simulink model "DynamicModel"  (R2018a)
settings: Solver=VariableStepAuto  StartTime=0.0  StopTime=10.0  RelTol=1e-3
model workspace (MAT data in the model file):
  Iz = 0.05807429185
  cf = 50000
  cr = 50000
  k1 = 2
  k2 = 5
  k3 = 3
  k4 = 6
  lf = 0.16002
  lr = 0.16002
  m = 2.26796
libraries: templibrary x1, dspmathops x1
settings Model: Creator=aswerdlow  LastModifiedBy=aswerdlow

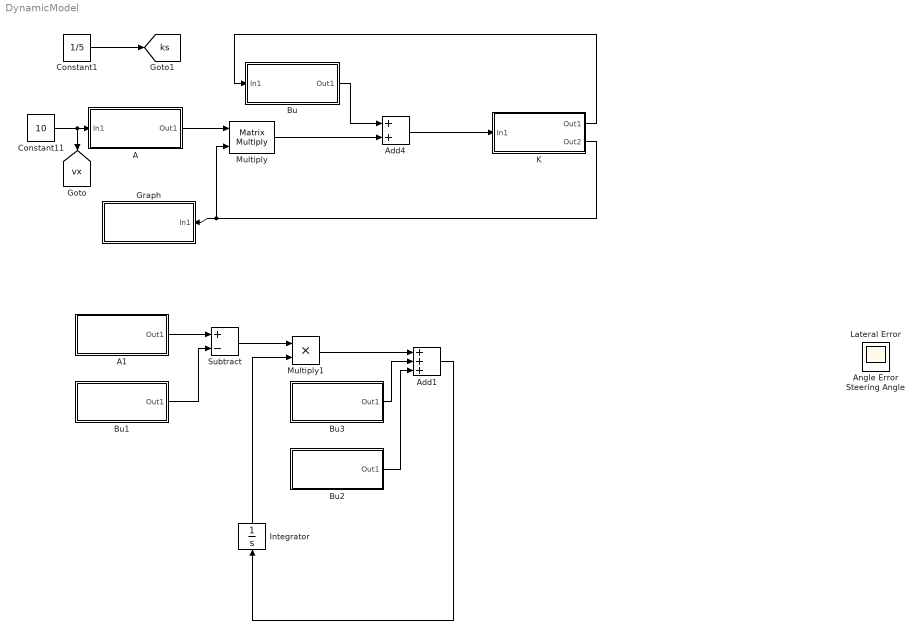
== system DynamicModel ==
  A : Subsystem
  A1 : Subsystem
  Add1 : Sum  Inputs=+++
  Add4 : Sum
  Bu : Subsystem
  Bu1 : Subsystem
  Bu2 : Subsystem
  Bu3 : Subsystem
  Constant1 : Constant  Value=1/5
  Constant11 : Constant  Value=10
  Graph : Subsystem
  Integrator : Integrator
  K : Subsystem
  Multiply : Product  Multiplication=Matrix(*)
  Multiply1 : Product
  Subtract : Sum  Inputs=+-
  Angle Error : Scope
  Lateral Error : Scope
  Steering Angle : Scope
  tag scope: ks=global, vx=global
  wires:
  Constant11/1 -> A/1(In1), [vx]
  A/1(Out1) -> Multiply/1
  Multiply/1 -> Add4/2
  Bu/1(Out1) -> Add4/1
  Add4/1 -> K/1(In1)
  K/1(Out1) -> Bu/1(In1)
  K/2(Out2) -> Graph/1(In1), Multiply/2
  Constant1/1 -> [ks]
  Subtract/1 -> Multiply1/1
  Bu1/1(Out1) -> Subtract/2
  Multiply1/1 -> Add1/1
  Integrator/1 -> Multiply1/2
  Add1/1 -> Integrator/1
  Bu3/1(Out1) -> Add1/2
  Bu2/1(Out1) -> Add1/3
  A1/1(Out1) -> Subtract/1

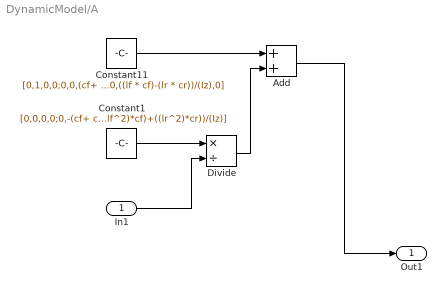
== system DynamicModel/A ==
  In1 : Inport
  Add : Sum
  Constant1 : Constant  Value=[0,0,0,0;0,-(cf+ cr)/(m),0,(lr * cr)-(lf * cf)/(m);0,0,0,0;0,((lr * cr)-(lf * cf))/(Iz),0,-(((lf^2)*cf)+((lr^2)*cr))/(Iz)]  VectorParams1D=off
  Constant11 : Constant  Value=[0,1,0,0;0,0,(cf+ cr)/(m),0;0,0,0,1;0,0,((lf * cf)-(lr * cr))/(Iz),0]  VectorParams1D=off
  Divide : Product  Inputs=*/
  Out1 : Outport
  wires:
  In1/1 -> Divide/2
  Constant11/1 -> Add/1
  Constant1/1 -> Divide/1
  Divide/1 -> Add/2
  Add/1 -> Out1/1

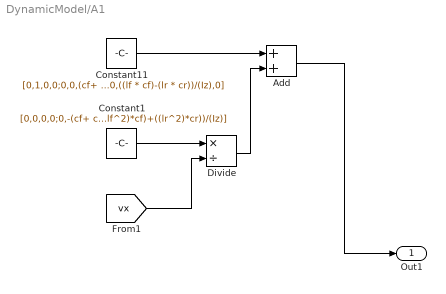
== system DynamicModel/A1 ==
  Add : Sum
  Constant1 : Constant  Value=[0,0,0,0;0,-(cf+ cr)/(m),0,(lr * cr)-(lf * cf)/(m);0,0,0,0;0,((lr * cr)-(lf * cf))/(Iz),0,-(((lf^2)*cf)+((lr^2)*cr))/(Iz)]  VectorParams1D=off
  Constant11 : Constant  Value=[0,1,0,0;0,0,(cf+ cr)/(m),0;0,0,0,1;0,0,((lf * cf)-(lr * cr))/(Iz),0]  VectorParams1D=off
  Divide : Product  Inputs=*/
  Out1 : Outport
  wires:
  [vx] -> Divide/2
  Constant11/1 -> Add/1
  Constant1/1 -> Divide/1
  Divide/1 -> Add/2
  Add/1 -> Out1/1

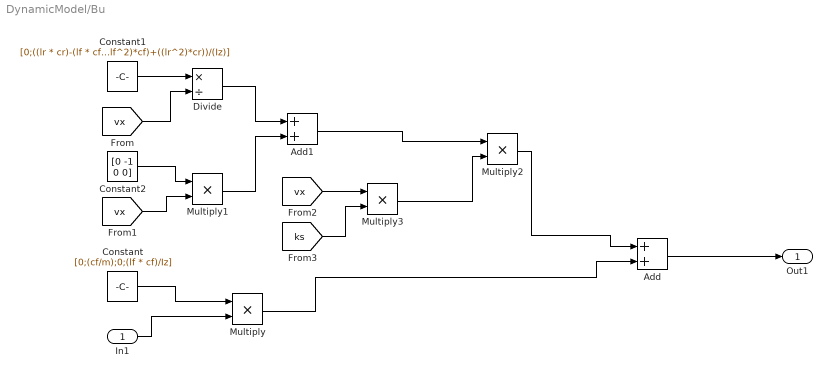
== system DynamicModel/Bu ==
  In1 : Inport
  Add : Sum
  Add1 : Sum
  Constant : Constant  Value=[0;(cf/m);0;(lf * cf)/Iz]  VectorParams1D=off
  Constant1 : Constant  Value=[0;((lr * cr)-(lf * cf))/m;0;-(((lf^2)*cf)+((lr^2)*cr))/(Iz)]  VectorParams1D=off
  Constant2 : Constant  Value=[0 -1 0 0]
  Divide : Product  Inputs=*/
  Multiply{,1..3} (4 alike) : Product
  Out1 : Outport
  wires:
  In1/1 -> Multiply/2
  Add/1 -> Out1/1
  Constant/1 -> Multiply/1
  Multiply/1 -> Add/2
  Constant1/1 -> Divide/1
  [vx] -> Divide/2
  Constant2/1 -> Multiply1/1
  [vx] -> Multiply1/2
  Divide/1 -> Add1/1
  Multiply1/1 -> Add1/2
  Add1/1 -> Multiply2/1
  [vx] -> Multiply3/1
  [ks] -> Multiply3/2
  Multiply3/1 -> Multiply2/2
  Multiply2/1 -> Add/1

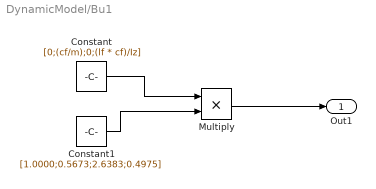
== system DynamicModel/Bu1 ==
  Constant : Constant  Value=[0;(cf/m);0;(lf * cf)/Iz]  VectorParams1D=off
  Constant1 : Constant  Value=[1.0000;0.5673;2.6383;0.4975]  VectorParams1D=off
  Multiply : Product
  Out1 : Outport
  wires:
  Constant1/1 -> Multiply/2
  Multiply/1 -> Out1/1
  Constant/1 -> Multiply/1

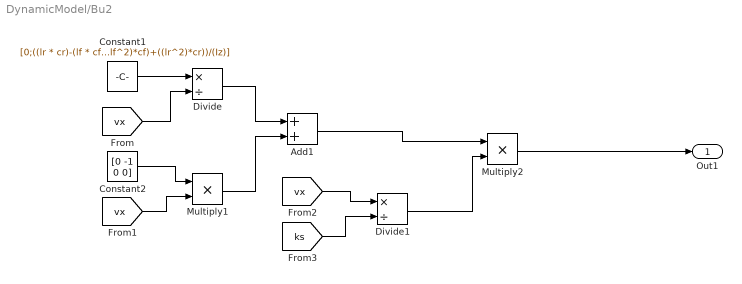
== system DynamicModel/Bu2 ==
  Add1 : Sum
  Constant1 : Constant  Value=[0;((lr * cr)-(lf * cf))/m;0;-(((lf^2)*cf)+((lr^2)*cr))/(Iz)]  VectorParams1D=off
  Constant2 : Constant  Value=[0 -1 0 0]
  Divide : Product  Inputs=*/
  Divide1 : Product  Inputs=*/
  Multiply1 : Product
  Multiply2 : Product
  Out1 : Outport
  wires:
  Multiply2/1 -> Out1/1
  Constant1/1 -> Divide/1
  [vx] -> Divide/2
  Constant2/1 -> Multiply1/1
  [vx] -> Multiply1/2
  Divide/1 -> Add1/1
  Multiply1/1 -> Add1/2
  Add1/1 -> Multiply2/1
  [vx] -> Divide1/1
  [ks] -> Divide1/2
  Divide1/1 -> Multiply2/2

== system DynamicModel/Bu3 ==
  Constant : Constant  Value=[0;(cf/m);0;(lf * cf)/Iz]  VectorParams1D=off
  Multiply : Product
  Subsystem : Subsystem
  Out1 : Outport
  wires:
  Multiply/1 -> Out1/1
  Constant/1 -> Multiply/1
  Subsystem/1(Out1) -> Multiply/2

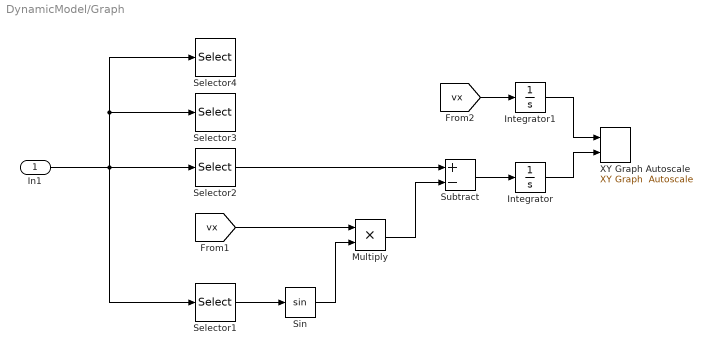
== system DynamicModel/Graph ==
  In1 : Inport
  Integrator : Integrator
  Integrator1 : Integrator
  Multiply : Product
  Selector1 : Selector  InputPortWidth=4  IndexOptions=Index vector (dialog)  Indices=3  OutputSizes=1
  Selector2 : Selector  InputPortWidth=4  IndexOptions=Index vector (dialog)  Indices=2  OutputSizes=1
  Selector3 : Selector  InputPortWidth=4  IndexOptions=Index vector (dialog)  Indices=3  OutputSizes=1
  Selector4 : Selector  InputPortWidth=4  IndexOptions=Index vector (dialog)  Indices=1  OutputSizes=1
  Sin : Trigonometry
  Subtract : Sum  Inputs=+-
  XY Graph Autoscale : templibrary/XY Graph  Autoscale  xmin=-1  xmax=1  ymin=-1  ymax=1  st=-1
  wires:
  Selector2/1 -> Subtract/1
  In1/1 -> Selector3/1, Selector4/1, Selector2/1, Selector1/1
  [vx] -> Multiply/1
  Sin/1 -> Multiply/2
  Selector1/1 -> Sin/1
  Multiply/1 -> Subtract/2
  Subtract/1 -> Integrator/1
  [vx] -> Integrator1/1
  Integrator1/1 -> XY Graph Autoscale/1
  Integrator/1 -> XY Graph Autoscale/2

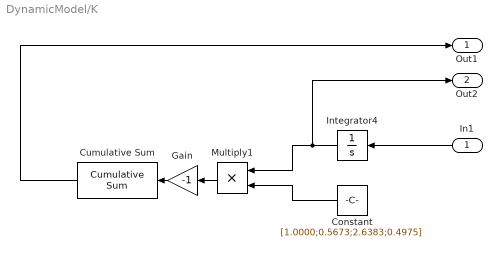
== system DynamicModel/K ==
  In1 : Inport
  Constant : Constant  Value=[1.0000;0.5673;2.6383;0.4975]  VectorParams1D=off
  Cumulative Sum : dspmathops/Cumulative Sum  dim=Columns  InputProcessing=Columns as channels (frame based)  reset_popup=None  roundingMode=Floor  overflowMode=off  outputDataTypeStr=Inherit: Same as accumulator  outputMin=[]  outputMax=[]  outputLastDataTypeStr=Inherit: Same as accumulator
      settings: SourceProductName=DSP System Toolbox
  Gain : Gain  Gain=-1
  Integrator4 : Integrator
  Multiply1 : Product
  Out1 : Outport
  Out2 : Outport  Port=2
  wires:
  In1/1 -> Integrator4/1
  Cumulative Sum/1 -> Out1/1
  Integrator4/1 -> Out2/1, Multiply1/1
  Constant/1 -> Multiply1/2
  Multiply1/1 -> Gain/1
  Gain/1 -> Cumulative Sum/1

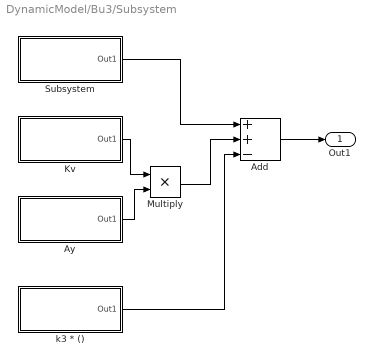
== system DynamicModel/Bu3/Subsystem ==
  Add : Sum  Inputs=++-
  Ay : Subsystem
  Kv : Subsystem
  Multiply : Product
  Subsystem : Subsystem
  k3 * () : Subsystem
  Out1 : Outport
  wires:
  Kv/1(Out1) -> Multiply/1
  Ay/1(Out1) -> Multiply/2
  Multiply/1 -> Add/2
  Add/1 -> Out1/1
  k3 * ()/1(Out1) -> Add/3
  Subsystem/1(Out1) -> Add/1

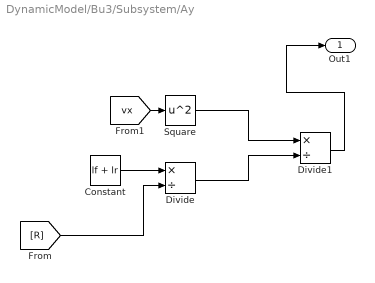
== system DynamicModel/Bu3/Subsystem/Ay ==
  Constant : Constant  Value=lf + lr
  Divide : Product  Inputs=*/
  Divide1 : Product  Inputs=*/
  Square : Math  Operator=square  SaturateOnIntegerOverflow=on
  Out1 : Outport
  wires:
  Constant/1 -> Divide/1
  [R] -> Divide/2
  Square/1 -> Divide1/1
  Divide/1 -> Divide1/2
  [vx] -> Square/1
  Divide1/1 -> Out1/1

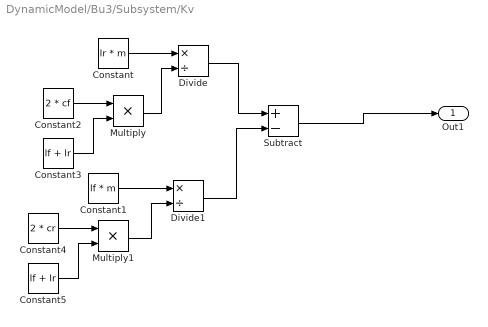
== system DynamicModel/Bu3/Subsystem/Kv ==
  Constant : Constant  Value=lr * m
  Constant1 : Constant  Value=lf * m
  Constant2 : Constant  Value=2 * cf
  Constant3 : Constant  Value=lf + lr
  Constant4 : Constant  Value=2 * cr
  Constant5 : Constant  Value=lf + lr
  Divide : Product  Inputs=*/
  Divide1 : Product  Inputs=*/
  Multiply : Product
  Multiply1 : Product
  Subtract : Sum  Inputs=+-
  Out1 : Outport
  wires:
  Divide/1 -> Subtract/1
  Divide1/1 -> Subtract/2
  Constant/1 -> Divide/1
  Constant1/1 -> Divide1/1
  Constant2/1 -> Multiply/1
  Constant3/1 -> Multiply/2
  Multiply/1 -> Divide/2
  Constant5/1 -> Multiply1/2
  Constant4/1 -> Multiply1/1
  Multiply1/1 -> Divide1/2
  Subtract/1 -> Out1/1

== system DynamicModel/Bu3/Subsystem/Subsystem ==
  Divide : Product  Inputs=*/
  Out1 : Outport
  wires:
  [L] -> Divide/1
  Divide/1 -> Out1/1
  [R] -> Divide/2

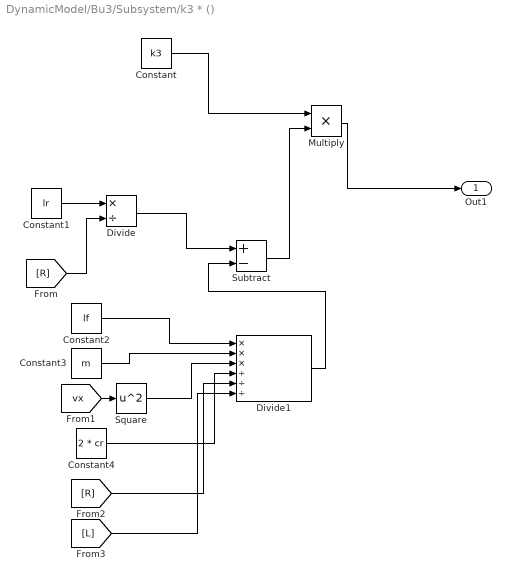
== system DynamicModel/Bu3/Subsystem/k3 * () ==
  Constant : Constant  Value=k3
  Constant1 : Constant  Value=lr
  Constant2 : Constant  Value=lf
  Constant3 : Constant  Value=m
  Constant4 : Constant  Value=2 * cr
  Divide : Product  Inputs=*/
  Divide1 : Product  Inputs=***///
  Multiply : Product
  Square : Math  Operator=square  SaturateOnIntegerOverflow=on
  Subtract : Sum  Inputs=+-
  Out1 : Outport
  wires:
  Constant/1 -> Multiply/1
  Multiply/1 -> Out1/1
  Divide/1 -> Subtract/1
  Constant1/1 -> Divide/1
  [R] -> Divide/2
  Divide1/1 -> Subtract/2
  Constant2/1 -> Divide1/1
  Constant3/1 -> Divide1/2
  [vx] -> Square/1
  Square/1 -> Divide1/3
  Constant4/1 -> Divide1/4
  [R] -> Divide1/5
  [L] -> Divide1/6
  Subtract/1 -> Multiply/2
